simulink model "SF007A_SysFricLrng"  (R2013b)
settings: Solver=FixedStepDiscrete  SolverMode=SingleTasking  StartTime=0.0  StopTime=1  FixedStep=0.002  RelTol=1e-3
PostLoadFcn:
  | , if any(exist('dsrtsu_mdlpostloadfcn', 'file') == [2, 3, 6]), try dsrtsu_mdlpostloadfcn('Execute', bdroot); catch fprintf('Error in PostLoadFcn (dsrtsu_mdlpostloadfcn) for model "%s":\n %s\n', bdroot, lasterr); end, end,
values from neighbouring files (symbols this model uses):
  ARCHGLBPRM_100MILLISEC_SEC_F32 = DataDict.Constant    [SF007A_SysFricLrng_DataDict.m]
  ARCHGLBPRM_10MILLISEC_SEC_F32 = DataDict.Constant    [SF007A_SysFricLrng_DataDict.m]
  ARCHGLBPRM_180OVERPI_ULS_F32 = DataDict.Constant    [SF007A_SysFricLrng_DataDict.m]
  CONV100MICROSECTOSEC_ULS_F32 = DataDict.Constant    [SF007A_SysFricLrng_DataDict.m]
  FLTINJ_SYSFRICLRNG_SYSFRICOFFS = DataDict.Constant    [SF007A_SysFricLrng_DataDict.m]
  FricLrngData = DataDict.NVM    [SF007A_SysFricLrng_DataDict.m]
  HWPTNUM_CNT_U08 = DataDict.Constant    [SF007A_SysFricLrng_DataDict.m]
  HWPTNUMSUB1_CNT_U08 = DataDict.Constant    [SF007A_SysFricLrng_DataDict.m]
  HWVELDECDIR_ULS_U08 = DataDict.Constant    [SF007A_SysFricLrng_DataDict.m]
  HWVELINCDIR_ULS_U08 = DataDict.Constant    [SF007A_SysFricLrng_DataDict.m]
  IDXCALCNSCAGFAC_ULS_U08 = DataDict.Constant    [SF007A_SysFricLrng_DataDict.m]
  IDXSELN1_ULS_U08 = DataDict.Constant    [SF007A_SysFricLrng_DataDict.m]
  IDXSELN2_ULS_U08 = DataDict.Constant    [SF007A_SysFricLrng_DataDict.m]
  IDXSELN3_ULS_U08 = DataDict.Constant    [SF007A_SysFricLrng_DataDict.m]
  LRNGENASCAFAC_MILLISEC_U32 = DataDict.Constant    [SF007A_SysFricLrng_DataDict.m]
  SCAGFACQUARTER_CNT_F32 = DataDict.Constant    [SF007A_SysFricLrng_DataDict.m]
  SCAGFACTEN_CNT_U16 = DataDict.Constant    [SF007A_SysFricLrng_DataDict.m]
  SCAGFACVEHLATA_MTRPERSECSQD_F32 = DataDict.Constant    [SF007A_SysFricLrng_DataDict.m]
  SECIDXSELN_ULS_U08 = DataDict.Constant    [SF007A_SysFricLrng_DataDict.m]
  SysFricLrngBasLineEolFric = DataDict.Calibration    [SF007A_SysFricLrng_DataDict.m]
  SysFricLrngBasLineFric = DataDict.Calibration    [SF007A_SysFricLrng_DataDict.m]
  SysFricLrngBasLineHys = DataDict.Calibration    [SF007A_SysFricLrng_DataDict.m]
  SysFricLrngBasLineRngCntr = DataDict.Calibration    [SF007A_SysFricLrng_DataDict.m]
  SysFricLrngEolFricDifScagFac = DataDict.Calibration    [SF007A_SysFricLrng_DataDict.m]
  SysFricLrngFricChgWght = DataDict.Calibration    [SF007A_SysFricLrng_DataDict.m]
  SysFricLrngFricDiagcThd = DataDict.Calibration    [SF007A_SysFricLrng_DataDict.m]
  SysFricLrngFricDiagcTiThd = DataDict.Calibration    [SF007A_SysFricLrng_DataDict.m]
  SysFricLrngFricHysHwAgPt = DataDict.Calibration    [SF007A_SysFricLrng_DataDict.m]
  SysFricLrngGain = DataDict.Calibration    [SF007A_SysFricLrng_DataDict.m]
  SysFricLrngHwPosnAuthyThd = DataDict.Calibration    [SF007A_SysFricLrng_DataDict.m]
  SysFricLrngHwVelConstrLim = DataDict.Calibration    [SF007A_SysFricLrng_DataDict.m]
  SysFricLrngHwVelHiLim = DataDict.Calibration    [SF007A_SysFricLrng_DataDict.m]
  SysFricLrngHwVelLoLim = DataDict.Calibration    [SF007A_SysFricLrng_DataDict.m]
  SysFricLrngIgnCycFricChgLim = DataDict.Calibration    [SF007A_SysFricLrng_DataDict.m]
  SysFricLrngLatAHiLim = DataDict.Calibration    [SF007A_SysFricLrng_DataDict.m]
  SysFricLrngLatALoLim = DataDict.Calibration    [SF007A_SysFricLrng_DataDict.m]
  SysFricLrngMaskVehSpd = DataDict.Calibration    [SF007A_SysFricLrng_DataDict.m]
  SysFricLrngRngCntrThd = DataDict.Calibration    [SF007A_SysFricLrng_DataDict.m]
  SysFricLrngThd = DataDict.Calibration    [SF007A_SysFricLrng_DataDict.m]
  SysFricLrngTHiLim = DataDict.Calibration    [SF007A_SysFricLrng_DataDict.m]
  SysFricLrngTLoLim = DataDict.Calibration    [SF007A_SysFricLrng_DataDict.m]
  SysFricLrngVehSpd = DataDict.Calibration    [SF007A_SysFricLrng_DataDict.m]
  SYSFRICOFFSLIM_HWNWTMTR_F32 = DataDict.Constant    [SF007A_SysFricLrng_DataDict.m]
  VEHSPDPTNUM1_ULS_U08 = DataDict.Constant    [SF007A_SysFricLrng_DataDict.m]
  VEHSPDPTNUM2_ULS_U08 = DataDict.Constant    [SF007A_SysFricLrng_DataDict.m]
undefined symbols (not defined in the file or in its folder): NtcNr1, NtcSts1, SysFricLrngOperMod1
libraries: Fil x19, simulink x17, NxtrLim x10, NxtrAbslt x3, NxtrNvM x2, FixdToFloat x2, FloatToFixd x1, LnrIntrpn x1
(part 6 of 7)

== system SF007A_SysFricLrng/SysFricLrng/SysFricLrngPer1/RunningAndCalibrationModes/FricLearning/Calculate Average Friction/NTC FAIL/GetTiSpan100MicroSec32bit ==
  note: Subtract original reference time
  note: seconds
  note: microseconds
  note: counts
  note: Wrap-to-zero
  note: 1 count = 100 uSec
  note: Get current system time
  note: GetTiSpan100MicroSec32bit
  note: Created Aug 18, 2015
      | Modified Oct 21, 2015
      | Modified Oct 30, 2015
      | Kevin Derry
  RefTmr : Inport
  CopyRight2 : Subsystem  Description=|  mask(Copyright Information){none=on}
      | Copyright info block.                                               
      |                                                                     
      | Place copyright information at the top of every subsystem in design.
      mask prompts: none "No parameters"
      mask help: Place copyright information at the top of every subsystem in design.
      mask Display:
      | NxtrConf = 'Nexteer Confidential';
      | 
      | sys = bdroot; %handle for the current model ("system")
      | first = get_param(sys,'Created');
      | if(isempty(first))
      |     first = datestr(now,'yyyy');
      | else
      |     first = first(end-3:end);  %year is last four digits
      | end
      | 
      | last = get_param(sys,'LastModifiedDate');
      | if isempty(last)
      |     last = datestr(now,'yyyy');
      | else
      |     last = last(end-3:end);
      | end
      | 
      | if strcmp(first,last)
      |     fprintf('%s -- Copyright %s Nexteer',NxtrConf,first)
      | else
      |     fprintf('%s -- %s%s- %s Nexteer',NxtrConf,char(169),first,last)
      | end
  Count per uSec : Constant  Value=0.01
  Data Store Read1 : DataStoreRead  DataStoreName=SimnTi
  Data Type Conversion2 : DataTypeConversion  OutDataTypeStr=uint32
  Divide1 : Product  Inputs=**
  Divide2 : Product  Inputs=*/
  If : If  NumInputs=2  IfExpression=u1 >= u2
  Max Counts : Constant  Value=2^32-1
  Merge : Merge
  No wrapping : Subsystem  TreatAsAtomicUnit=on
  Product2 : Product
  Product3 : Product
  Rounding : Rounding
  Subtract3 : Sum  Inputs=+-
  Wrapping : Subsystem  TreatAsAtomicUnit=on
  uSec per Sec : Constant  Value=1000000
  TiSpan : Outport
  wires:
  Wrapping/1(Out1) -> Merge/2
  No wrapping/1(Out1) -> Merge/1
  If/2 -> Wrapping/Action
  If/1 -> No wrapping/Action
  Product3/1 -> Subtract3/2
  Subtract3/1 -> Data Type Conversion2/1
  Rounding/1 -> Product3/1
  Divide2/1 -> Rounding/1
  Max Counts/1 -> Divide2/2, Product3/2
  Divide1/1 -> Divide2/1, Subtract3/1
  Product2/1 -> Divide1/1
  Data Store Read1/1 -> Product2/1
  Count per uSec/1 -> Divide1/2
  uSec per Sec/1 -> Product2/2
  Merge/1 -> TiSpan/1
  RefTmr/1 -> If/2, No wrapping/2(ref), Wrapping/2(ref)
  Data Type Conversion2/1 -> If/1, No wrapping/1(new), Wrapping/1(new)

== system SF007A_SysFricLrng/SysFricLrng/SysFricLrngPer1/RunningAndCalibrationModes/FricLearning/Calculate Average Friction/NTC FAIL/NTCFAIL ==
  NtcNr : Inport
  NtcStInfo : Inport  Port=2
  NtcSts : Inport  Port=3
  DebStep : Inport  Port=4
  Action Port : ActionPort  ActionType=then
  CopyRight2 : Subsystem  Description=|  mask(Copyright Information){none=on}
      | Copyright info block.                                               
      |                                                                     
      | Place copyright information at the top of every subsystem in design.
      mask prompts: none "No parameters"
      mask help: Place copyright information at the top of every subsystem in design.
      mask Display:
      | NxtrConf = 'Nexteer Confidential';
      | 
      | sys = bdroot; %handle for the current model ("system")
      | first = get_param(sys,'Created');
      | first = first(end-3:end);  %year is last four digits
      | 
      | last = get_param(sys,'LastModifiedDate');
      | if isempty(last)
      |     last = datestr(now,'yyyy');
      | else
      |     last = last(end-3:end);
      | end
      | 
      | if strcmp(first,last)
      |     fprintf('%s -- Copyright %s Nexteer',NxtrConf,first)
      | else
      |     fprintf('%s -- %s%s- %s Nexteer',NxtrConf,char(169),first,last)
      | end
  SetNtcSts : Subsystem  mask(SetNTC){}
      mask help: SetNTC library block
  wires:
  NtcStInfo/1 -> SetNtcSts/2(NtcStInfo)
  NtcSts/1 -> SetNtcSts/3(NtcSts)
  DebStep/1 -> SetNtcSts/4(DebStep)
  NtcNr/1 -> SetNtcSts/1(NtcNr)

== system SF007A_SysFricLrng/SysFricLrng/SysFricLrngPer1/RunningAndCalibrationModes/FricLearning/Calculate Average Friction/NTC PASS /CopyRight2 ==

== system SF007A_SysFricLrng/SysFricLrng/SysFricLrngPer1/RunningAndCalibrationModes/FricLearning/Calculate Average Friction/NTC PASS /GetRefTmr100MicroSec32bit ==
  note: 1 count = 100 uSec
  note: seconds
  note: microseconds
  note: counts
  note: Wrap-to-zero
  note: GetRefTmr100MicroSec32bit
  note: Created Aug 18, 2015
      | Modified Oct 21, 2015
      | Modified Oct 30, 2015
      | Kevin Derry
  CopyRight2 : Subsystem  Description=|  mask(Copyright Information){none=on}
      | Copyright info block.                                               
      |                                                                     
      | Place copyright information at the top of every subsystem in design.
      mask prompts: none "No parameters"
      mask help: Place copyright information at the top of every subsystem in design.
      mask Display:
      | NxtrConf = 'Nexteer Confidential';
      | 
      | sys = bdroot; %handle for the current model ("system")
      | first = get_param(sys,'Created');
      | if(isempty(first))
      |     first = datestr(now,'yyyy');
      | else
      |     first = first(end-3:end);  %year is last four digits
      | end
      | 
      | last = get_param(sys,'LastModifiedDate');
      | if isempty(last)
      |     last = datestr(now,'yyyy');
      | else
      |     last = last(end-3:end);
      | end
      | 
      | if strcmp(first,last)
      |     fprintf('%s -- Copyright %s Nexteer',NxtrConf,first)
      | else
      |     fprintf('%s -- %s%s- %s Nexteer',NxtrConf,char(169),first,last)
      | end
  Count per uSec : Constant  Value=0.01
  Data Store Read1 : DataStoreRead  DataStoreName=SimnTi
  Data Type Conversion1 : DataTypeConversion  OutDataTypeStr=uint32
  Divide1 : Product  Inputs=**
  Divide2 : Product  Inputs=*/
  Max Counts : Constant  Value=2^32-1
  Product1 : Product
  Product2 : Product
  Rounding : Rounding
  Subtract1 : Sum  Inputs=+-
  uSec per Sec : Constant  Value=1000000
  RefTmr : Outport
  wires:
  Product2/1 -> Subtract1/2
  Subtract1/1 -> Data Type Conversion1/1
  Rounding/1 -> Product2/1
  Divide2/1 -> Rounding/1
  Max Counts/1 -> Divide2/2, Product2/2
  Divide1/1 -> Divide2/1, Subtract1/1
  Product1/1 -> Divide1/1
  Count per uSec/1 -> Divide1/2
  uSec per Sec/1 -> Product1/2
  Data Type Conversion1/1 -> RefTmr/1
  Data Store Read1/1 -> Product1/1

== system SF007A_SysFricLrng/SysFricLrng/SysFricLrngPer1/RunningAndCalibrationModes/FricLearning/Calculate Average Friction/NTC PASS /SetNtcSts ==
  NtcNr : Inport
  NtcStInfo : Inport  Port=2
  NtcSts : Inport  Port=3
  DebStep : Inport  Port=4
  Data Type Conversion : DataTypeConversion
  SetNtcSts : Subsystem  TreatAsAtomicUnit=on
      settings: RTWSystemCode=Inline
  wires:
  NtcStInfo/1 -> SetNtcSts/2(NtcStInfo)
  DebStep/1 -> Data Type Conversion/1
  NtcSts/1 -> SetNtcSts/3(NtcSts)
  NtcNr/1 -> SetNtcSts/1(NtcNr)  "NtcNr"
  Data Type Conversion/1 -> SetNtcSts/4(DebStep)

== system SF007A_SysFricLrng/SysFricLrng/SysFricLrngPer1/RunningAndCalibrationModes/FricLearning/Calculate Average Friction/Raw Average Calculation/CopyRight2 ==

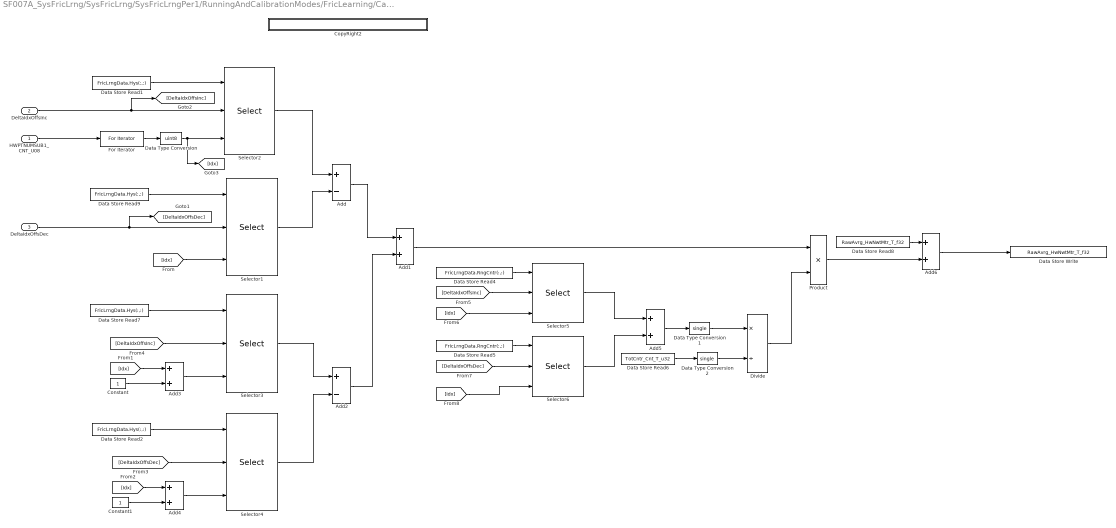
== system SF007A_SysFricLrng/SysFricLrng/SysFricLrngPer1/RunningAndCalibrationModes/FricLearning/Calculate Average Friction/Raw Average Calculation/Raw Average ==
  HWPTNUMSUB1_CNT_U08 : Inport
  DeltaIdxOffsInc : Inport  Port=2
  DeltaIdxOffsDec : Inport  Port=3
  Add : Sum  Inputs=+-
  Add{1,3..6} (5 alike) : Sum
  Add2 : Sum  Inputs=+-
  Constant : Constant  OutDataTypeStr=uint8
      settings: AttributesFormatString=%<OutDataTypeStr>
  Constant1 : Constant  OutDataTypeStr=uint8
      settings: AttributesFormatString=%<OutDataTypeStr>
  CopyRight2 : Subsystem  Description=|  mask(Copyright Information){none=on}
      | Copyright info block.                                               
      |                                                                     
      | Place copyright information at the top of every subsystem in design.
      mask prompts: none "No parameters"
      mask help: Place copyright information at the top of every subsystem in design.
      mask Display:
      | NxtrConf = 'Nexteer Confidential';
      | 
      | sys = bdroot; %handle for the current model ("system")
      | first = get_param(sys,'Created');
      | first = first(end-3:end);  %year is last four digits
      | 
      | last = get_param(sys,'LastModifiedDate');
      | if isempty(last)
      |     last = datestr(now,'yyyy');
      | else
      |     last = last(end-3:end);
      | end
      | 
      | if strcmp(first,last)
      |     fprintf('%s -- Copyright %s Nexteer',NxtrConf,first)
      | else
      |     fprintf('%s -- %s%s- %s Nexteer',NxtrConf,char(169),first,last)
      | end
  Data Store Read{1..2,7,9} (4 alike) : DataStoreRead  Priority=1  DataStoreName=FricLrngData  DataStoreElements=FricLrngData.Hys(:,:)
      settings: AttributesFormatString=Priority: %<Priority>
  Data Store Read4 : DataStoreRead  Priority=1  DataStoreName=FricLrngData  DataStoreElements=FricLrngData.RngCntr(:,:)
      settings: AttributesFormatString=Priority:%<Priority>
  Data Store Read5 : DataStoreRead  Priority=1  DataStoreName=FricLrngData  DataStoreElements=FricLrngData.RngCntr(:,:)
      settings: AttributesFormatString=Priority:%<Priority>
  Data Store Read6 : DataStoreRead  Priority=1  DataStoreName=TotCntr_Cnt_T_u32
      settings: AttributesFormatString=Priority:%<Priority>
  Data Store Read8 : DataStoreRead  Priority=1  DataStoreName=RawAvrg_HwNwtMtr_T_f32
      settings: AttributesFormatString=Priority:%<Priority>
  Data Store Write : DataStoreWrite  Priority=2  DataStoreName=RawAvrg_HwNwtMtr_T_f32
      settings: AttributesFormatString=Priority:%<Priority>
  Data Type Conversion : DataTypeConversion  OutDataTypeStr=uint8
  Data Type Conversion1 : DataTypeConversion  OutDataTypeStr=single
  Data Type Conversion2 : DataTypeConversion  OutDataTypeStr=single
  Divide : Product  Inputs=*/
  For Iterator : ForIterator  IterationSource=external  IterationVariableDataType=int8
  Product : Product
  Selector{1..6} (6 alike) : Selector  NumberOfDimensions=2  InputPortWidth=4  IndexOptions=Index vector (port),Index vector (port)  Indices=[1 3],1  OutputSizes=1,1
  wires:
  Data Store Read9/1 -> Selector1/1
  DeltaIdxOffsDec/1 -> Selector1/2, [DeltaIdxOffsDec]
  DeltaIdxOffsInc/1 -> [DeltaIdxOffsInc], Selector2/2
  [Idx] -> Selector1/3
  Data Store Read1/1 -> Selector2/1
  For Iterator/1 -> Data Type Conversion/1
  Selector2/1 -> Add/1
  Selector1/1 -> Add/2
  Add/1 -> Add1/1
  Data Store Read2/1 -> Selector4/1
  Data Store Read7/1 -> Selector3/1
  [DeltaIdxOffsDec] -> Selector4/2
  [DeltaIdxOffsInc] -> Selector3/2
  Add2/1 -> Add1/2
  Selector3/1 -> Add2/1
  Selector4/1 -> Add2/2
  [Idx] -> Add3/1
  Add3/1 -> Selector3/3
  Data Type Conversion/1 -> Selector2/3, [Idx]
  [Idx] -> Add4/1
  Constant/1 -> Add3/2
  Constant1/1 -> Add4/2
  Add4/1 -> Selector4/3
  Data Store Read4/1 -> Selector5/1
  Add1/1 -> Product/1
  Data Store Read5/1 -> Selector6/1
  [DeltaIdxOffsInc] -> Selector5/2
  [Idx] -> Selector5/3
  [DeltaIdxOffsDec] -> Selector6/2
  [Idx] -> Selector6/3
  Selector6/1 -> Add5/2
  Add5/1 -> Data Type Conversion1/1
  Data Store Read6/1 -> Data Type Conversion2/1
  Data Store Read8/1 -> Add6/1
  Add6/1 -> Data Store Write/1
  HWPTNUMSUB1_CNT_U08/1 -> For Iterator/1
  Divide/1 -> Product/2
  Product/1 -> Add6/2
  Selector5/1 -> Add5/1
  Data Type Conversion1/1 -> Divide/1
  Data Type Conversion2/1 -> Divide/2

== system SF007A_SysFricLrng/SysFricLrng/SysFricLrngPer1/RunningAndCalibrationModes/FricLearning/Calculate Average Friction/Raw Average Calculation/Update LPF ==
  RawAvrg_HwNwtMtr_T_f32 : Inport
  VehSpdIndex : Inport  Port=2
  Assignment4 : Assignment  IndexOptions=Index vector (port)  Indices=1  OutputSizes=1
  CopyRight2 : Subsystem  Description=|  mask(Copyright Information){none=on}
      | Copyright info block.                                               
      |                                                                     
      | Place copyright information at the top of every subsystem in design.
      mask prompts: none "No parameters"
      mask help: Place copyright information at the top of every subsystem in design.
      mask Display:
      | NxtrConf = 'Nexteer Confidential';
      | 
      | sys = bdroot; %handle for the current model ("system")
      | first = get_param(sys,'Created');
      | first = first(end-3:end);  %year is last four digits
      | 
      | last = get_param(sys,'LastModifiedDate');
      | if isempty(last)
      |     last = datestr(now,'yyyy');
      | else
      |     last = last(end-3:end);
      | end
      | 
      | if strcmp(first,last)
      |     fprintf('%s -- Copyright %s Nexteer',NxtrConf,first)
      | else
      |     fprintf('%s -- %s%s- %s Nexteer',NxtrConf,char(169),first,last)
      | end
  Data Store Read1 : DataStoreRead  Priority=1  DataStoreName=FilAvrgFric
  Data Store Write1 : DataStoreWrite  Priority=2  DataStoreName=FilAvrgFric
  InitAvrgFricLpFil1 : Subsystem
  InitAvrgFricLpFil2 : Subsystem
  InitAvrgFricLpFil3 : Subsystem
  InitAvrgFricLpFil4 : Subsystem
  Merge : Merge  Inputs=4
  Switch Case : SwitchCase  CaseConditions={1, 2, 3}
  FiltAvgFric : Outport
  wires:
  Assignment4/1 -> Data Store Write1/1
  Data Store Read1/1 -> Assignment4/1
  RawAvrg_HwNwtMtr_T_f32/1 -> [RawAvgFric]
  VehSpdIndex/1 -> [VehSpdIdx], Assignment4/3
  [RawAvgFric] -> InitAvrgFricLpFil1/1(RawAvgFric)
  [VehSpdIdx] -> Switch Case/1
  Switch Case/1 -> InitAvrgFricLpFil1/Action
  Switch Case/2 -> InitAvrgFricLpFil2/Action
  Switch Case/3 -> InitAvrgFricLpFil3/Action
  Switch Case/4 -> InitAvrgFricLpFil4/Action
  InitAvrgFricLpFil1/1(FiltAvgFric) -> Merge/1
  InitAvrgFricLpFil2/1(FiltAvgFric) -> Merge/2
  InitAvrgFricLpFil3/1(FiltAvgFric) -> Merge/3
  InitAvrgFricLpFil4/1(FiltAvgFric) -> Merge/4
  [RawAvgFric] -> InitAvrgFricLpFil2/1(RawAvgFric)
  [RawAvgFric] -> InitAvrgFricLpFil3/1(RawAvgFric)
  [RawAvgFric] -> InitAvrgFricLpFil4/1(RawAvgFric)
  Merge/1 -> Assignment4/2, FiltAvgFric/1

== system SF007A_SysFricLrng/SysFricLrng/SysFricLrngPer1/RunningAndCalibrationModes/FricLearning/Calculate Average Friction/Total Counter Updation/CopyRight2 ==

== system SF007A_SysFricLrng/SysFricLrng/SysFricLrngPer1/RunningAndCalibrationModes/FricLearning/Range Counter Manager/Range Counter Control/CopyRight2 ==

== system SF007A_SysFricLrng/SysFricLrng/SysFricLrngPer1/RunningAndCalibrationModes/FricLearning/Range Counter Manager/Range Counter Control1/CopyRight2 ==

== system SF007A_SysFricLrng/SysFricLrng/SysFricLrngPer1/RunningAndCalibrationModes/FricLearning/Range Counter Manager/Range Counter Control1/UpdateBaselineFric ==
  HWPTNUMSUB1_CNT_U08 : Inport
  DeltaIdxOffsInc : Inport  Port=2
  DeltaIdxOffsDec : Inport  Port=3
  Assignment : Assignment  NumberOfDimensions=2  IndexOptions=Index vector (port),Index vector (port)  Indices=1,1  OutputSizes=1,1
  Assignment1 : Assignment  NumberOfDimensions=2  IndexOptions=Index vector (port),Index vector (port)  Indices=1,1  OutputSizes=1,1
  Constant1 : Constant  Value=SCAGFACTEN_CNT_U16
  Constant3 : Constant  Value=SCAGFACTEN_CNT_U16
  CopyRight2 : Subsystem  Description=|  mask(Copyright Information){none=on}
      | Copyright info block.                                               
      |                                                                     
      | Place copyright information at the top of every subsystem in design.
      mask prompts: none "No parameters"
      mask help: Place copyright information at the top of every subsystem in design.
      mask Display:
      | NxtrConf = 'Nexteer Confidential';
      | 
      | sys = bdroot; %handle for the current model ("system")
      | first = get_param(sys,'Created');
      | first = first(end-3:end);  %year is last four digits
      | 
      | last = get_param(sys,'LastModifiedDate');
      | if isempty(last)
      |     last = datestr(now,'yyyy');
      | else
      |     last = last(end-3:end);
      | end
      | 
      | if strcmp(first,last)
      |     fprintf('%s -- Copyright %s Nexteer',NxtrConf,first)
      | else
      |     fprintf('%s -- %s%s- %s Nexteer',NxtrConf,char(169),first,last)
      | end
  Data Store Read1 : DataStoreRead  Priority=1  DataStoreName=FricLrngData  DataStoreElements=FricLrngData.RngCntr(:,:)
      settings: AttributesFormatString=Priority:%<Priority>
  Data Store Read7 : DataStoreRead  Priority=1  DataStoreName=FricLrngData  DataStoreElements=FricLrngData.RngCntr(:,:)
      settings: AttributesFormatString=Priority:%<Priority>
  Data Store Write1 : DataStoreWrite  Priority=2  DataStoreName=FricLrngData  DataStoreElements=FricLrngData.RngCntr(:,:)
      settings: AttributesFormatString=Priority:%<Priority>
  Data Store Write8 : DataStoreWrite  Priority=2  DataStoreName=FricLrngData  DataStoreElements=FricLrngData.RngCntr(:,:)
      settings: AttributesFormatString=Priority:%<Priority>
  Divide : Product  Inputs=*/
  Divide1 : Product  Inputs=*/
  For Iterator : ForIterator  IterationSource=external  IterationVariableDataType=int8
  Selector1 : Selector  NumberOfDimensions=2  InputPortWidth=4  IndexOptions=Index vector (port),Index vector (port)  Indices=[1 3],1  OutputSizes=1,1
  Selector2 : Selector  NumberOfDimensions=2  InputPortWidth=4  IndexOptions=Index vector (port),Index vector (port)  Indices=[1 3],1  OutputSizes=1,1
  wires:
  Data Store Read7/1 -> Assignment/1, Selector1/1
  HWPTNUMSUB1_CNT_U08/1 -> For Iterator/1
  For Iterator/1 -> Selector1/3, [Idx]
  DeltaIdxOffsDec/1 -> [DeltaIdxOffsDec], Selector1/2
  Selector1/1 -> Divide/1
  Divide/1 -> Assignment/2
  DeltaIdxOffsInc/1 -> [DeltaIdxOffsInc], Selector2/2
  [Idx] -> Selector2/3
  [Idx] -> Assignment1/4
  [Idx] -> Assignment/4
  [DeltaIdxOffsDec] -> Assignment/3
  [DeltaIdxOffsInc] -> Assignment1/3
  Selector2/1 -> Divide1/1
  Divide1/1 -> Assignment1/2
  Data Store Read1/1 -> Assignment1/1, Selector2/1
  Constant1/1 -> Divide/2
  Constant3/1 -> Divide1/2
  Assignment/1 -> Data Store Write8/1
  Assignment1/1 -> Data Store Write1/1

== system SF007A_SysFricLrng/SysFricLrng/SysFricLrngPer1/RunningAndCalibrationModes/FricLearning/Range Counter Manager/Range Counter Threshold Calculation/CopyRight2 ==

== system SF007A_SysFricLrng/SysFricLrng/SysFricLrngPer1/RunningAndCalibrationModes/FricLearning/Range Counter Manager/Range Counter Threshold Calculation/Do Nothig ==
  Action Port : ActionPort  ActionType=else
  CopyRight2 : Subsystem  Description=|  mask(Copyright Information){none=on}
      | Copyright info block.                                               
      |                                                                     
      | Place copyright information at the top of every subsystem in design.
      mask prompts: none "No parameters"
      mask help: Place copyright information at the top of every subsystem in design.
      mask Display:
      | NxtrConf = 'Nexteer Confidential';
      | 
      | sys = bdroot; %handle for the current model ("system")
      | first = get_param(sys,'Created');
      | first = first(end-3:end);  %year is last four digits
      | 
      | last = get_param(sys,'LastModifiedDate');
      | if isempty(last)
      |     last = datestr(now,'yyyy');
      | else
      |     last = last(end-3:end);
      | end
      | 
      | if strcmp(first,last)
      |     fprintf('%s -- Copyright %s Nexteer',NxtrConf,first)
      | else
      |     fprintf('%s -- %s%s- %s Nexteer',NxtrConf,char(169),first,last)
      | end

== system SF007A_SysFricLrng/SysFricLrng/SysFricLrngPer1/RunningAndCalibrationModes/FricLearning/Range Counter Manager/Range Counter Threshold Calculation/RangeCounterThreshExceeded ==
  Action Port : ActionPort  ActionType=then
  Constant1 : Constant  OutDataTypeStr=boolean
  CopyRight2 : Subsystem  Description=|  mask(Copyright Information){none=on}
      | Copyright info block.                                               
      |                                                                     
      | Place copyright information at the top of every subsystem in design.
      mask prompts: none "No parameters"
      mask help: Place copyright information at the top of every subsystem in design.
      mask Display:
      | NxtrConf = 'Nexteer Confidential';
      | 
      | sys = bdroot; %handle for the current model ("system")
      | first = get_param(sys,'Created');
      | first = first(end-3:end);  %year is last four digits
      | 
      | last = get_param(sys,'LastModifiedDate');
      | if isempty(last)
      |     last = datestr(now,'yyyy');
      | else
      |     last = last(end-3:end);
      | end
      | 
      | if strcmp(first,last)
      |     fprintf('%s -- Copyright %s Nexteer',NxtrConf,first)
      | else
      |     fprintf('%s -- %s%s- %s Nexteer',NxtrConf,char(169),first,last)
      | end
  Data Store Write1 : DataStoreWrite  Priority=1  DataStoreName=RngCntrThdExcdd_Cnt_T_lgc
      settings: AttributesFormatString=Priority:%<Priority>
  wires:
  Constant1/1 -> Data Store Write1/1

== system SF007A_SysFricLrng/SysFricLrng/SysFricLrngPer1/RunningAndCalibrationModes/LearningConstraint/ColTqconstraint/ColTqAryCalcn/12 Delay's Execution ==
  Add : Sum  Inputs=+-
  Add1 : Sum  Inputs=+-
  Assignment : Assignment  IndexOptions=Index vector (port)  Indices=1  OutputSizes=1
  Constant1 : Constant  Value=IDXSELN2_ULS_U08
  Constant2 : Constant  Value=IDXSELN1_ULS_U08
  CopyRight2 : Subsystem  Description=|  mask(Copyright Information){none=on}
      | Copyright info block.                                               
      |                                                                     
      | Place copyright information at the top of every subsystem in design.
      mask prompts: none "No parameters"
      mask help: Place copyright information at the top of every subsystem in design.
      mask Display:
      | NxtrConf = 'Nexteer Confidential';
      | 
      | sys = bdroot; %handle for the current model ("system")
      | first = get_param(sys,'Created');
      | first = first(end-3:end);  %year is last four digits
      | 
      | last = get_param(sys,'LastModifiedDate');
      | if isempty(last)
      |     last = datestr(now,'yyyy');
      | else
      |     last = last(end-3:end);
      | end
      | 
      | if strcmp(first,last)
      |     fprintf('%s -- Copyright %s Nexteer',NxtrConf,first)
      | else
      |     fprintf('%s -- %s%s- %s Nexteer',NxtrConf,char(169),first,last)
      | end
  Data Store Read : DataStoreRead  DataStoreName=ColTqAry
  Data Store Read1 : DataStoreRead  DataStoreName=ColTqAry
  Data Store Write : DataStoreWrite  DataStoreName=ColTqAry
  For Iterator : ForIterator  IterationLimit=11
  Selector : Selector  InputPortWidth=12  IndexOptions=Index vector (port)  Indices=[1]  OutputSizes=1
  wires:
  Data Store Read/1 -> Assignment/1
  Assignment/1 -> Data Store Write/1
  Selector/1 -> Assignment/2
  Constant1/1 -> Add/1
  Data Store Read1/1 -> Selector/1
  Constant2/1 -> Add1/1
  Add1/1 -> Selector/2
  Add/1 -> Assignment/3
  For Iterator/1 -> Add1/2, Add/2

== system SF007A_SysFricLrng/SysFricLrng/SysFricLrngPer1/RunningAndCalibrationModes/LearningConstraint/ColTqconstraint/ColTqAryCalcn/CopyRight2 ==

== system SF007A_SysFricLrng/SysFricLrng/SysFricLrngPer1/RunningAndCalibrationModes/LearningConstraint/Get System Time/GetRefTmr100MicroSec32bit/CopyRight2 ==

== system SF007A_SysFricLrng/SysFricLrng/SysFricLrngPer1/RunningAndCalibrationModes/LearningConstraint/GetTiSpan100MicroSec32bit/No wrapping/CopyRight2 ==

== system SF007A_SysFricLrng/SysFricLrng/SysFricLrngPer1/RunningAndCalibrationModes/LearningConstraint/GetTiSpan100MicroSec32bit/Wrapping/CopyRight2 ==

== system SF007A_SysFricLrng/SysFricLrng/SysFricLrngPer1/RunningAndCalibrationModes/LearningConstraint/HwAngConstraint/Handwheel Angle Buffer/12 Delay's Execution ==
  Add : Sum  Inputs=+-
  Add1 : Sum  Inputs=+-
  Assignment : Assignment  IndexOptions=Index vector (port)  Indices=1  OutputSizes=1
  Constant1 : Constant  Value=IDXSELN2_ULS_U08
  Constant2 : Constant  Value=IDXSELN1_ULS_U08
  CopyRight2 : Subsystem  Description=|  mask(Copyright Information){none=on}
      | Copyright info block.                                               
      |                                                                     
      | Place copyright information at the top of every subsystem in design.
      mask prompts: none "No parameters"
      mask help: Place copyright information at the top of every subsystem in design.
      mask Display:
      | NxtrConf = 'Nexteer Confidential';
      | 
      | sys = bdroot; %handle for the current model ("system")
      | first = get_param(sys,'Created');
      | first = first(end-3:end);  %year is last four digits
      | 
      | last = get_param(sys,'LastModifiedDate');
      | if isempty(last)
      |     last = datestr(now,'yyyy');
      | else
      |     last = last(end-3:end);
      | end
      | 
      | if strcmp(first,last)
      |     fprintf('%s -- Copyright %s Nexteer',NxtrConf,first)
      | else
      |     fprintf('%s -- %s%s- %s Nexteer',NxtrConf,char(169),first,last)
      | end
  Data Store Read : DataStoreRead  DataStoreName=HwAgBuf
  Data Store Read1 : DataStoreRead  DataStoreName=HwAgBuf
  Data Store Write : DataStoreWrite  DataStoreName=HwAgBuf
  For Iterator : ForIterator  IterationLimit=11
  Selector : Selector  InputPortWidth=12  IndexOptions=Index vector (port)  Indices=[1]  OutputSizes=1
  wires:
  Data Store Read/1 -> Assignment/1
  Assignment/1 -> Data Store Write/1
  Selector/1 -> Assignment/2
  Constant1/1 -> Add/1
  Data Store Read1/1 -> Selector/1
  Constant2/1 -> Add1/1
  Add1/1 -> Selector/2
  Add/1 -> Assignment/3
  For Iterator/1 -> Add1/2, Add/2

== system SF007A_SysFricLrng/SysFricLrng/SysFricLrngPer1/RunningAndCalibrationModes/LearningConstraint/HwAngConstraint/Handwheel Angle Buffer/CopyRight2 ==

== system SF007A_SysFricLrng/SysFricLrng/SysFricLrngPer1/RunningAndCalibrationModes/LearningConstraint/HwVelConstraint/Decreasing Direction/CopyRight2 ==

== system SF007A_SysFricLrng/SysFricLrng/SysFricLrngPer1/RunningAndCalibrationModes/LearningConstraint/HwVelConstraint/Handwheel Velocity Buffer/12 Delay's Execution ==
  note: Create a buffer of 12(IDXSELN1_ULS_U08) Hw Velocity values.
      | All 12 values must lie between the min and max values of calibration table.
      | Otuput a Hw Velocity value from the middle of buffer and a flag to indicate whether all buffered points met the requirment.
  Add : Sum  Inputs=+-
  Add1 : Sum  Inputs=+-
  Assignment : Assignment  IndexOptions=Index vector (port)  Indices=1  OutputSizes=1
  Constant1 : Constant  Value=IDXSELN2_ULS_U08
  Constant2 : Constant  Value=IDXSELN1_ULS_U08
  CopyRight2 : Subsystem  Description=|  mask(Copyright Information){none=on}
      | Copyright info block.                                               
      |                                                                     
      | Place copyright information at the top of every subsystem in design.
      mask prompts: none "No parameters"
      mask help: Place copyright information at the top of every subsystem in design.
      mask Display:
      | NxtrConf = 'Nexteer Confidential';
      | 
      | sys = bdroot; %handle for the current model ("system")
      | first = get_param(sys,'Created');
      | first = first(end-3:end);  %year is last four digits
      | 
      | last = get_param(sys,'LastModifiedDate');
      | if isempty(last)
      |     last = datestr(now,'yyyy');
      | else
      |     last = last(end-3:end);
      | end
      | 
      | if strcmp(first,last)
      |     fprintf('%s -- Copyright %s Nexteer',NxtrConf,first)
      | else
      |     fprintf('%s -- %s%s- %s Nexteer',NxtrConf,char(169),first,last)
      | end
  Data Store Read : DataStoreRead  DataStoreName=HwVelBuf
  Data Store Read1 : DataStoreRead  DataStoreName=HwVelBuf
  Data Store Write : DataStoreWrite  DataStoreName=HwVelBuf
  For Iterator : ForIterator  IterationLimit=11
  Selector : Selector  InputPortWidth=12  IndexOptions=Index vector (port)  Indices=[1]  OutputSizes=1
  wires:
  Data Store Read/1 -> Assignment/1
  Assignment/1 -> Data Store Write/1
  Selector/1 -> Assignment/2
  Constant1/1 -> Add/1
  Data Store Read1/1 -> Selector/1
  Constant2/1 -> Add1/1
  Add1/1 -> Selector/2
  Add/1 -> Assignment/3
  For Iterator/1 -> Add1/2, Add/2

== system SF007A_SysFricLrng/SysFricLrng/SysFricLrngPer1/RunningAndCalibrationModes/LearningConstraint/HwVelConstraint/Handwheel Velocity Buffer/CopyRight2 ==

== system SF007A_SysFricLrng/SysFricLrng/SysFricLrngPer1/RunningAndCalibrationModes/LearningConstraint/HwVelConstraint/Increasing Direction/CopyRight2 ==

== system SF007A_SysFricLrng/SysFricLrng/SysFricLrngPer1/RunningAndCalibrationModes/LearningConstraint/HwVelConstraint/Increasing Direction/CopyRight2 ==

== system SF007A_SysFricLrng/SysFricLrng/SysFricLrngPer1/RunningAndCalibrationModes/LearningConstraint/HwVelConstraint/Range_Monotonicity Calculation/ AllGTZ ==
  Enable : EnablePort
  Constant1 : Constant  Value=false  OutDataTypeStr=boolean
      settings: AttributesFormatString=%<OutDataTypeStr>
  CopyRight2 : Subsystem  Description=|  mask(Copyright Information){none=on}
      | Copyright info block.                                               
      |                                                                     
      | Place copyright information at the top of every subsystem in design.
      mask prompts: none "No parameters"
      mask help: Place copyright information at the top of every subsystem in design.
      mask Display:
      | NxtrConf = 'Nexteer Confidential';
      | 
      | sys = bdroot; %handle for the current model ("system")
      | first = get_param(sys,'Created');
      | first = first(end-3:end);  %year is last four digits
      | 
      | last = get_param(sys,'LastModifiedDate');
      | if isempty(last)
      |     last = datestr(now,'yyyy');
      | else
      |     last = last(end-3:end);
      | end
      | 
      | if strcmp(first,last)
      |     fprintf('%s -- Copyright %s Nexteer',NxtrConf,first)
      | else
      |     fprintf('%s -- %s%s- %s Nexteer',NxtrConf,char(169),first,last)
      | end
  Data Store Write1 : DataStoreWrite  Priority=1  DataStoreName=VariPosRng_Cnt_T_lgc
      settings: AttributesFormatString=Priority:%<Priority>
  wires:
  Constant1/1 -> Data Store Write1/1

== system SF007A_SysFricLrng/SysFricLrng/SysFricLrngPer1/RunningAndCalibrationModes/LearningConstraint/HwVelConstraint/Range_Monotonicity Calculation/AllLTZ ==
  Enable : EnablePort
  Constant1 : Constant  Value=false  OutDataTypeStr=boolean
      settings: AttributesFormatString=%<OutDataTypeStr>
  CopyRight2 : Subsystem  Description=|  mask(Copyright Information){none=on}
      | Copyright info block.                                               
      |                                                                     
      | Place copyright information at the top of every subsystem in design.
      mask prompts: none "No parameters"
      mask help: Place copyright information at the top of every subsystem in design.
      mask Display:
      | NxtrConf = 'Nexteer Confidential';
      | 
      | sys = bdroot; %handle for the current model ("system")
      | first = get_param(sys,'Created');
      | first = first(end-3:end);  %year is last four digits
      | 
      | last = get_param(sys,'LastModifiedDate');
      | if isempty(last)
      |     last = datestr(now,'yyyy');
      | else
      |     last = last(end-3:end);
      | end
      | 
      | if strcmp(first,last)
      |     fprintf('%s -- Copyright %s Nexteer',NxtrConf,first)
      | else
      |     fprintf('%s -- %s%s- %s Nexteer',NxtrConf,char(169),first,last)
      | end
  Data Store Write1 : DataStoreWrite  Priority=1  DataStoreName=VariNegRng_Cnt_T_lgc
      settings: AttributesFormatString=Priority:%<Priority>
  wires:
  Constant1/1 -> Data Store Write1/1

== system SF007A_SysFricLrng/SysFricLrng/SysFricLrngPer1/RunningAndCalibrationModes/LearningConstraint/HwVelConstraint/Range_Monotonicity Calculation/CopyRight2 ==

== system SF007A_SysFricLrng/SysFricLrng/SysFricLrngPer1/RunningAndCalibrationModes/LearningConstraint/VehSpdConstraint/VehSpdIdxCalcn/CopyRight2 ==

== system SF007A_SysFricLrng/SysFricLrng/SysFricLrngPer1/RunningAndCalibrationModes/Running Mode/If Action Subsystem/BlendingFricChg/CopyRight2 ==

== system SF007A_SysFricLrng/SysFricLrng/SysFricLrngPer1/RunningAndCalibrationModes/Running Mode/If Action Subsystem/BlendingFricChg/FilLpUpdOutp ==
  Input : Inport
  Add : Sum
  Data Store Read : DataStoreRead  DataStoreName=FricChgLpFil  DataStoreElements=FricChgLpFil.FilSt#FricChgLpFil.FilGain
  Data Store Write : DataStoreWrite  DataStoreName=FricChgLpFil  DataStoreElements=FricChgLpFil.FilSt
  Product : Product
  Subtract : Sum  Inputs=+-
  Out1 : Outport  OutDataTypeStr=single
  wires:
  Data Store Read/2 -> Product/2
  Add/1 -> Out1/1, Data Store Write/1
  Product/1 -> Add/2
  Subtract/1 -> Product/1
  Input/1 -> Subtract/1
  Data Store Read/1 -> Subtract/2, Add/1

== system SF007A_SysFricLrng/SysFricLrng/SysFricLrngPer1/RunningAndCalibrationModes/FricLearning/Calculate Average Friction/Max Raw Average Calculation/MaxRawAvrg/CopyRight2 ==

== system SF007A_SysFricLrng/SysFricLrng/SysFricLrngPer1/RunningAndCalibrationModes/FricLearning/Calculate Average Friction/NTC FAIL/Do Nothing/CopyRight2 ==

== system SF007A_SysFricLrng/SysFricLrng/SysFricLrngPer1/RunningAndCalibrationModes/FricLearning/Calculate Average Friction/NTC FAIL/GetTiSpan100MicroSec32bit/CopyRight2 ==

== system SF007A_SysFricLrng/SysFricLrng/SysFricLrngPer1/RunningAndCalibrationModes/FricLearning/Calculate Average Friction/NTC FAIL/GetTiSpan100MicroSec32bit/No wrapping ==
  new : Inport
  ref : Inport  Port=2
  Action Port : ActionPort  ActionType=then
  CopyRight2 : Subsystem  Description=|  mask(Copyright Information){none=on}
      | Copyright info block.                                               
      |                                                                     
      | Place copyright information at the top of every subsystem in design.
      mask prompts: none "No parameters"
      mask help: Place copyright information at the top of every subsystem in design.
      mask Display:
      | NxtrConf = 'Nexteer Confidential';
      | 
      | sys = bdroot; %handle for the current model ("system")
      | first = get_param(sys,'Created');
      | if(isempty(first))
      |     first = datestr(now,'yyyy');
      | else
      |     first = first(end-3:end);  %year is last four digits
      | end
      | 
      | last = get_param(sys,'LastModifiedDate');
      | if isempty(last)
      |     last = datestr(now,'yyyy');
      | else
      |     last = last(end-3:end);
      | end
      | 
      | if strcmp(first,last)
      |     fprintf('%s -- Copyright %s Nexteer',NxtrConf,first)
      | else
      |     fprintf('%s -- %s%s- %s Nexteer',NxtrConf,char(169),first,last)
      | end
  Subtract1 : Sum  Inputs=+-
  Out1 : Outport
  wires:
  ref/1 -> Subtract1/2
  new/1 -> Subtract1/1
  Subtract1/1 -> Out1/1

== system SF007A_SysFricLrng/SysFricLrng/SysFricLrngPer1/RunningAndCalibrationModes/FricLearning/Calculate Average Friction/NTC FAIL/GetTiSpan100MicroSec32bit/Wrapping ==
  new : Inport
  ref : Inport  Port=2
  Action Port : ActionPort  ActionType=else
  CopyRight2 : Subsystem  Description=|  mask(Copyright Information){none=on}
      | Copyright info block.                                               
      |                                                                     
      | Place copyright information at the top of every subsystem in design.
      mask prompts: none "No parameters"
      mask help: Place copyright information at the top of every subsystem in design.
      mask Display:
      | NxtrConf = 'Nexteer Confidential';
      | 
      | sys = bdroot; %handle for the current model ("system")
      | first = get_param(sys,'Created');
      | if(isempty(first))
      |     first = datestr(now,'yyyy');
      | else
      |     first = first(end-3:end);  %year is last four digits
      | end
      | 
      | last = get_param(sys,'LastModifiedDate');
      | if isempty(last)
      |     last = datestr(now,'yyyy');
      | else
      |     last = last(end-3:end);
      | end
      | 
      | if strcmp(first,last)
      |     fprintf('%s -- Copyright %s Nexteer',NxtrConf,first)
      | else
      |     fprintf('%s -- %s%s- %s Nexteer',NxtrConf,char(169),first,last)
      | end
  Max Counts : Constant  Value=2^32-1  OutDataTypeStr=uint32
  Subtract1 : Sum  Inputs=+-+
  Out1 : Outport
  wires:
  new/1 -> Subtract1/3
  ref/1 -> Subtract1/2
  Max Counts/1 -> Subtract1/1
  Subtract1/1 -> Out1/1

== system SF007A_SysFricLrng/SysFricLrng/SysFricLrngPer1/RunningAndCalibrationModes/FricLearning/Calculate Average Friction/NTC FAIL/NTCFAIL/CopyRight2 ==

== system SF007A_SysFricLrng/SysFricLrng/SysFricLrngPer1/RunningAndCalibrationModes/FricLearning/Calculate Average Friction/NTC FAIL/NTCFAIL/SetNtcSts ==
  NtcNr : Inport
  NtcStInfo : Inport  Port=2
  NtcSts : Inport  Port=3
  DebStep : Inport  Port=4
  SetNtcSts : Subsystem  TreatAsAtomicUnit=on
      settings: RTWSystemCode=Inline
  wires:
  NtcNr/1 -> SetNtcSts/1(NtcNr)  "NtcNr"
  NtcSts/1 -> SetNtcSts/3(NtcSts)
  DebStep/1 -> SetNtcSts/4(DebStep)
  NtcStInfo/1 -> SetNtcSts/2(NtcStInfo)

== system SF007A_SysFricLrng/SysFricLrng/SysFricLrngPer1/RunningAndCalibrationModes/FricLearning/Calculate Average Friction/NTC PASS /GetRefTmr100MicroSec32bit/CopyRight2 ==

== system SF007A_SysFricLrng/SysFricLrng/SysFricLrngPer1/RunningAndCalibrationModes/FricLearning/Calculate Average Friction/NTC PASS /SetNtcSts/SetNtcSts ==
  note: Note:
      |
      | - "ISO Fault Debounce Design" Simulink block intent to use here for Simulation purpose only. Do not Code this block
  NtcNr : Inport
  NtcStInfo : Inport  Port=2
  NtcSts : Inport  Port=3
  DebStep : Inport  Port=4
  CopyRight2 : Subsystem  Description=|  mask(Copyright Information){none=on}
      | Copyright info block.                                               
      |                                                                     
      | Place copyright information at the top of every subsystem in design.
      mask prompts: none "No parameters"
      mask help: Place copyright information at the top of every subsystem in design.
      mask Display:
      | NxtrConf = 'Nexteer Confidential';
      | 
      | sys = bdroot; %handle for the current model ("system")
      | first = get_param(sys,'Created');
      | first = first(end-3:end);  %year is last four digits
      | 
      | last = get_param(sys,'LastModifiedDate');
      | if isempty(last)
      |     last = datestr(now,'yyyy');
      | else
      |     last = last(end-3:end);
      | end
      | 
      | if strcmp(first,last)
      |     fprintf('%s -- Copyright %s Nexteer',NxtrConf,first)
      | else
      |     fprintf('%s -- %s%s- %s Nexteer',NxtrConf,char(169),first,last)
      | end
  Data Store Write : DataStoreWrite  DataStoreName=Ntc0X0A2Qlfr
  Data Type Conversion4 : DataTypeConversion  OutDataTypeStr=Enum: SigQlfr1
  Ground : Ground
  ISO Fault Debounce Design : Stateflow chart  TreatAsAtomicUnit=on
      settings: AttributesFormatString=|
      | Simulation Purpose Only.
      | Do Not Code this block
      | Diagnostic Manager Owns this requirement
  Terminator : Terminator
  Terminator1 : Terminator
  wires:
  Ground/1 -> ISO Fault Debounce Design/3(SvcClr)
  DebStep/1 -> ISO Fault Debounce Design/2(DebStep)
  NtcSts/1 -> ISO Fault Debounce Design/1(NtcSts)
  NtcNr/1 -> Terminator/1
  NtcStInfo/1 -> Terminator1/1
  Data Type Conversion4/1 -> Data Store Write/1
  ISO Fault Debounce Design/1(Qualifier) -> Data Type Conversion4/1

== system SF007A_SysFricLrng/SysFricLrng/SysFricLrngPer1/RunningAndCalibrationModes/FricLearning/Calculate Average Friction/Raw Average Calculation/Raw Average/CopyRight2 ==

== system SF007A_SysFricLrng/SysFricLrng/SysFricLrngPer1/RunningAndCalibrationModes/FricLearning/Calculate Average Friction/Raw Average Calculation/Update LPF/CopyRight2 ==

== system SF007A_SysFricLrng/SysFricLrng/SysFricLrngPer1/RunningAndCalibrationModes/FricLearning/Calculate Average Friction/Raw Average Calculation/Update LPF/InitAvrgFricLpFil1 ==
  RawAvgFric : Inport
  Action Port : ActionPort  ActionType=case
  CopyRight2 : Subsystem  Description=|  mask(Copyright Information){none=on}
      | Copyright info block.                                               
      |                                                                     
      | Place copyright information at the top of every subsystem in design.
      mask prompts: none "No parameters"
      mask help: Place copyright information at the top of every subsystem in design.
      mask Display:
      | NxtrConf = 'Nexteer Confidential';
      | 
      | sys = bdroot; %handle for the current model ("system")
      | first = get_param(sys,'Created');
      | first = first(end-3:end);  %year is last four digits
      | 
      | last = get_param(sys,'LastModifiedDate');
      | if isempty(last)
      |     last = datestr(now,'yyyy');
      | else
      |     last = last(end-3:end);
      | end
      | 
      | if strcmp(first,last)
      |     fprintf('%s -- Copyright %s Nexteer',NxtrConf,first)
      | else
      |     fprintf('%s -- %s%s- %s Nexteer',NxtrConf,char(169),first,last)
      | end
  FilLpUpdOutp : Subsystem  mask(FilLpUpdOutp){StVar=AvrgFricLpFil1}
      mask prompts: StVar "State Variable:"
      mask help: Simulink implementation of the LPF_OpUpdate_f32_m macro.
      mask init: same as SF007A_SysFricLrng/SysFricLrng/SysFricLrngPer1/RunningAndCalibrationModes/Running Mode/If Action Subsystem/BlendingFricChg/FilLpUpdOutp
      settings: AttributesFormatString=StVar: %<StVar>
      mask Display:
      | port_label('input',1,'Inp')
      | port_label('output',1,'Outp')
      | text(0.2,0.8,'FilLpUpdOutp')
  FiltAvgFric : Outport
  wires:
  RawAvgFric/1 -> FilLpUpdOutp/1(Input)
  FilLpUpdOutp/1(Out1) -> FiltAvgFric/1

== system SF007A_SysFricLrng/SysFricLrng/SysFricLrngPer1/RunningAndCalibrationModes/FricLearning/Calculate Average Friction/Raw Average Calculation/Update LPF/InitAvrgFricLpFil2 ==
  RawAvgFric : Inport
  Action Port : ActionPort  ActionType=case
  CopyRight2 : Subsystem  Description=|  mask(Copyright Information){none=on}
      | Copyright info block.                                               
      |                                                                     
      | Place copyright information at the top of every subsystem in design.
      mask prompts: none "No parameters"
      mask help: Place copyright information at the top of every subsystem in design.
      mask Display:
      | NxtrConf = 'Nexteer Confidential';
      | 
      | sys = bdroot; %handle for the current model ("system")
      | first = get_param(sys,'Created');
      | first = first(end-3:end);  %year is last four digits
      | 
      | last = get_param(sys,'LastModifiedDate');
      | if isempty(last)
      |     last = datestr(now,'yyyy');
      | else
      |     last = last(end-3:end);
      | end
      | 
      | if strcmp(first,last)
      |     fprintf('%s -- Copyright %s Nexteer',NxtrConf,first)
      | else
      |     fprintf('%s -- %s%s- %s Nexteer',NxtrConf,char(169),first,last)
      | end
  FilLpUpdOutp : Subsystem  mask(FilLpUpdOutp){StVar=AvrgFricLpFil2}
      mask prompts: StVar "State Variable:"
      mask help: Simulink implementation of the LPF_OpUpdate_f32_m macro.
      mask init: same as SF007A_SysFricLrng/SysFricLrng/SysFricLrngPer1/RunningAndCalibrationModes/Running Mode/If Action Subsystem/BlendingFricChg/FilLpUpdOutp
      settings: AttributesFormatString=StVar: %<StVar>
      mask Display:
      | port_label('input',1,'Inp')
      | port_label('output',1,'Outp')
      | text(0.2,0.8,'FilLpUpdOutp')
  FiltAvgFric : Outport
  wires:
  RawAvgFric/1 -> FilLpUpdOutp/1(Input)
  FilLpUpdOutp/1(Out1) -> FiltAvgFric/1
